simulink model "wpr_spr_nl"  (Simulink 8.1)
settings: Solver=ode4  StartTime=0.0  StopTime=5.0  FixedStep=0.01  RelTol=1e-3
values from neighbouring files (symbols this model uses):
  h = 40    [2.mat]    (also in 3.mat)
  k = 200000    [3.mat]
  m = 14000    [3.mat]
  v0 = 70    [1.mat]    (also in 2.mat; 3.mat = 67)
settings Model: Creator=student  LastModifiedBy=adasdeb
settings DataIOCC: MaxDataPoints=100000  TimeSaveName=toutnl
settings DebuggingCC: FcnCallInpInsideContextMsg=EnableAllAsWarning
settings GRTTargetCC: CombineOutputUpdateFcns=on  GRTInterface=off

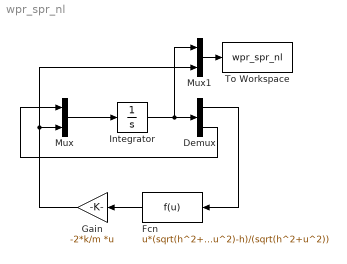
== system wpr_spr_nl ==
  Demux : Demux  Outputs=2
  Fcn : Fcn  Expr=u*(sqrt(h^2+u^2)-h)/(sqrt(h^2+u^2))
  Gain : Gain  Gain=-2*k/m  Multiplication=Matrix(K*u)
  Integrator : Integrator  InitialCondition=[0;v0]
  Mux : Mux  Inputs=2
  Mux1 : Mux  Inputs=2
  To Workspace : ToWorkspace  VariableName=wpr_spr_nl  SampleTime=-1
  wires:
  Demux/2 -> Mux/1
  Integrator/1 -> Mux1/1, Demux/1
  Mux/1 -> Integrator/1
  Demux/1 -> Fcn/1
  Gain/1 -> Mux/2, Mux1/2
  Fcn/1 -> Gain/1
  Mux1/1 -> To Workspace/1
